simulink model "heli_quanser_base_MC"  (R2025a)
settings: Solver=FixedStepAuto  StartTime=0.0  StopTime=15  FixedStep=0.001  RelTol=1e-3  EnableMultiTasking=on
values from neighbouring files (symbols this model uses):
  theta_0 = -40.5*pi/180    (= -0.706858347058)    [setup_heli_2d_base.m]
  Ts = 0.001    [setup_heli_2d_base.m]
  VMAX_UPM_P = 24    [setup_heli_2d_base.m]
  VMAX_UPM_Y = 15    [setup_heli_2d_base.m]
undefined symbols (not defined in the file or in its folder): B_p, B_y, g, J_eq_p, J_eq_y, K_pp, K_py, K_yp, K_yy, l_cm, m_heli
libraries: simulink x2, simulink_extras x1
settings Model: Creator=Jorge Romero  LastModifiedBy=440G5
settings SolverCC: AlgebraicLoopSolver=TrustRegion
settings DataIOCC: LimitDataPoints=on  SaveFormat=Array  ReturnWorkspaceOutputs=off
settings OptimizationCC: ExpressionDepthLimit=2147483647.0  LifeSpan=inf
settings DebuggingCC: UnderspecifiedInitializationDetection=Classic  MergeDetectMultiDrivingBlocksExec=none  SolverPrmCheckMsg=warning  UnconnectedInputMsg=warning  UnconnectedOutputMsg=warning  UnconnectedLineMsg=warning  StateNameClashWarn=warning  SFUnexpectedBacktrackingDiag=warning  SFNoUnconditionalDefaultTransitionDiag=warning  SFExecutionAtInitializationDiag=none  ArithmeticOperatorsInVariantConditions=warning
settings HardwareCC: ProdBitPerPointer=32.0  ProdBitPerSizeT=32.0  ProdBitPerPtrDiffT=32.0  ProdLargestAtomicFloat=None  ProdIntDivRoundTo=Undefined  ProdEndianess=Unspecified  ProdWordSize=32.0  ProdHWDeviceType=32-bit Generic
settings ModelReferenceCC: EnableRefExpFcnMdlSchedulingChecks=on  PropagateSignalLabelsOutOfModel=off
settings SFSimCC: SimUseLocalCustomCode=off  CustomCodeUndefinedFunction=UseInterfaceOnly
settings RTWCC: RTWUseLocalCustomCode=off  GPUComputeCapability=3.5  DLArmComputeVersion=19.05
settings CodeAppCC: StateflowObjectComments=on
settings GRTTargetCC: TargetLangStandard=C89/C90 (ANSI)
settings ConfigComp: CovMetricSettings=dw  CovSaveCumulativeToWorkspaceVar=on  CovSaveSingleToWorkspaceVar=on  CovExternalEMLEnable=off

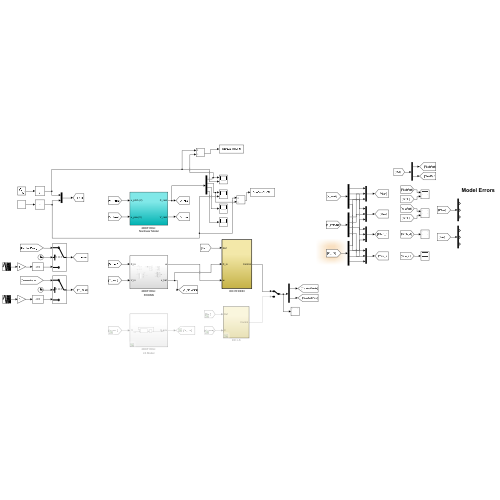
[thumbnail: Simulink's stored preview of the top-level diagram]
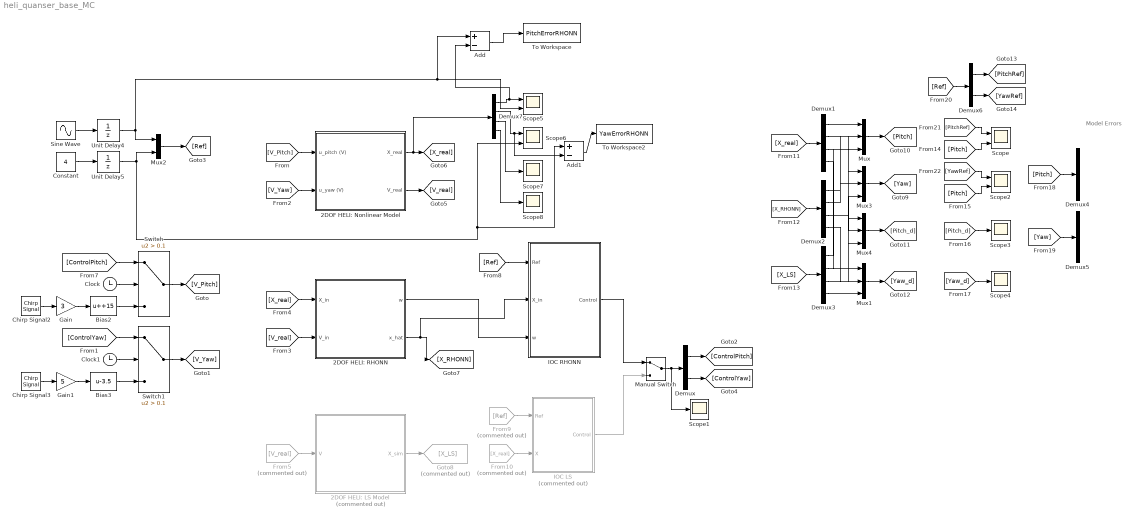
== system heli_quanser_base_MC ==
  note: Model Errors
  2DOF HELI: LS Model : Subsystem  Commented=on
  2DOF HELI: Nonlinear Model : Subsystem
  2DOF HELI: RHONN : Subsystem
  Add : Sum  Inputs=+-
  Add1 : Sum  Inputs=+-
  Bias2 : Bias  Bias=+15  SaturateOnIntegerOverflow=off
  Bias3 : Bias  Bias=-3.5  SaturateOnIntegerOverflow=off
  Chirp Signal2 : simulink/Sources/Chirp Signal  f1=0.08  T=10  f2=1
  Chirp Signal3 : simulink/Sources/Chirp Signal  f1=0.05  T=100  f2=1
  Clock : Clock
      settings: Decimation=5
  Clock1 : Clock
      settings: Decimation=5
  Constant : Constant  Value=4
  Demux : Demux  Outputs=2
  Demux{1..3,7} (4 alike) : Demux
  Demux4 : Demux  Outputs=3
  Demux5 : Demux  Outputs=3
  Demux6 : Demux  Outputs=2
  From10 : From  Commented=on  GotoTag=X_real
  From5 : From  Commented=on  GotoTag=V_real
  From9 : From  Commented=on  GotoTag=Ref
  Gain : Gain  Gain=3
  Gain1 : Gain  Gain=5
  Goto8 : Goto  Commented=on  GotoTag=X_LS
  IOC LS : Subsystem  Commented=on  TreatAsAtomicUnit=on
  IOC RHONN : Subsystem  TreatAsAtomicUnit=on
  Manual Switch : ManualSwitch
  Mux{,1,3..4} (4 alike) : Mux  Inputs=3
  Mux2 : Mux  Inputs=2
  Scope{,2,5..6} (4 alike) : Scope  NumInputPorts=2
      Scope settings: ActiveDisplayYMinimum=-2.2045251175704  ActiveDisplayYMaximum=12.772142587556569
      Scope2 settings: ActiveDisplayYMinimum=-2.2045251175704  ActiveDisplayYMaximum=12.772142587556569
      Scope5 settings: ActiveDisplayYMinimum=-1.4995166148869326  ActiveDisplayYMaximum=1.1943818734120628  DataLoggingVariableName=ScopeData4
      Scope6 settings: ActiveDisplayYMinimum=-31.385745513206732  ActiveDisplayYMaximum=23.73492677473369  DataLoggingVariableName=ScopeData5
  Scope{1,3..4,7..8} (5 alike) : Scope
      Scope1 settings: ActiveDisplayYMinimum=-26.503210929485832  ActiveDisplayYMaximum=16.085993128612095  DataLoggingVariableName=ScopeData14
      Scope3 settings: DataLoggingVariableName=ScopeData2
      Scope4 settings: DataLoggingVariableName=ScopeData3
      Scope7 settings: ActiveDisplayYMinimum=-2.2729284352396681  ActiveDisplayYMaximum=0.21801617430591014  DataLoggingVariableName=ScopeData6
      Scope8 settings: ActiveDisplayYMinimum=-1  ActiveDisplayYMaximum=1  DataLoggingVariableName=ScopeData7
  Sine Wave : Sin  Amplitude=0.45  SampleTime=0
  Switch : Switch  Criteria=u2 > Threshold  Threshold=0.1  SaturateOnIntegerOverflow=off  InputSameDT=off
  Switch1 : Switch  Criteria=u2 > Threshold  Threshold=0.1  SaturateOnIntegerOverflow=off  InputSameDT=off
  To Workspace : ToWorkspace  VariableName=PitchErrorRHONN  SaveFormat=Timeseries  SampleTime=-1
  To Workspace2 : ToWorkspace  VariableName=YawErrorRHONN  SaveFormat=Timeseries  SampleTime=-1
  Unit Delay4 : UnitDelay  SampleTime=-1  HasFrameUpgradeWarning=on
  Unit Delay5 : UnitDelay  SampleTime=-1  HasFrameUpgradeWarning=on
  wires:
  Gain/1 -> Bias2/1
  Bias2/1 -> Switch/3
  Chirp Signal2/1 -> Gain/1
  [ControlPitch] -> Switch/1
  Clock/1 -> Switch/2
  Bias3/1 -> Switch1/3
  Gain1/1 -> Bias3/1
  Clock1/1 -> Switch1/2
  Chirp Signal3/1 -> Gain1/1
  [ControlYaw] -> Switch1/1
  Switch/1 -> [V_Pitch]
  Switch1/1 -> [V_Yaw]
  [V_Pitch] -> 2DOF HELI: Nonlinear Model/1(u_pitch (V))
  [V_Yaw] -> 2DOF HELI: Nonlinear Model/2(u_yaw (V))
  From5/1 -> 2DOF HELI: LS Model/1(" V")
  IOC LS/1(Control) -> Manual Switch/2
  From9/1 -> IOC LS/1(Ref)
  Unit Delay4/1 -> Add/1, Scope5/2, Mux2/1
  Mux2/1 -> [Ref]
  Manual Switch/1 -> Scope1/1, Demux/1
  Demux/1 -> [ControlPitch]
  Demux/2 -> [ControlYaw]
  2DOF HELI: Nonlinear Model/2(V_real) -> [V_real]
  2DOF HELI: Nonlinear Model/1(X_real) -> Demux7/1, [X_real]
  From10/1 -> IOC LS/2(X)
  2DOF HELI: LS Model/1(X_sim) -> Goto8/1
  [X_RHONN] -> Demux2/1
  [X_real] -> Demux1/1
  [X_LS] -> Demux3/1
  Demux1/1 -> Mux/1
  Demux2/1 -> Mux/2
  Demux3/1 -> Mux/3
  Demux1/4 -> Mux1/1
  Demux2/4 -> Mux1/2
  Demux3/4 -> Mux1/3
  Demux1/2 -> Mux3/1
  Demux2/2 -> Mux3/2
  Demux3/2 -> Mux3/3
  Demux1/3 -> Mux4/1
  Demux2/3 -> Mux4/2
  Demux3/3 -> Mux4/3
  Mux/1 -> [Pitch]
  Mux3/1 -> [Yaw]
  Mux4/1 -> [Pitch_d]
  Mux1/1 -> [Yaw_d]
  [Pitch] -> Scope/2
  [Pitch_d] -> Scope3/1
  [Yaw_d] -> Scope4/1
  [Pitch] -> Demux4/1
  [Yaw] -> Demux5/1
  [Ref] -> Demux6/1
  [PitchRef] -> Scope/1
  [YawRef] -> Scope2/1
  [Pitch] -> Scope2/2
  Demux6/1 -> [PitchRef]
  Demux6/2 -> [YawRef]
  2DOF HELI: RHONN/2(x_hat) -> IOC RHONN/2(X_in), [X_RHONN]
  [X_real] -> 2DOF HELI: RHONN/1(X_in)
  [V_real] -> 2DOF HELI: RHONN/2(V_in)
  2DOF HELI: RHONN/1(w) -> IOC RHONN/3(w)
  IOC RHONN/1(Control) -> Manual Switch/1
  [Ref] -> IOC RHONN/1(Ref)
  Sine Wave/1 -> Unit Delay4/1
  Constant/1 -> Unit Delay5/1
  Demux7/1 -> Add/2, Scope5/1
  Demux7/2 -> Add1/2, Scope6/1
  Demux7/3 -> Scope7/1
  Demux7/4 -> Scope8/1
  Add/1 -> To Workspace/1
  Unit Delay5/1 -> Mux2/2, Scope6/2, Add1/1
  Add1/1 -> To Workspace2/1

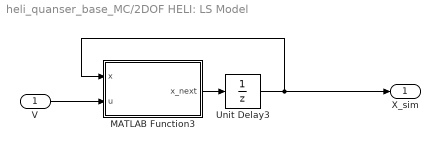
== system heli_quanser_base_MC/2DOF HELI: LS Model ==
  " V" : Inport
  MATLAB Function3 : MATLAB Function  TreatAsAtomicUnit=on
  Unit Delay3 : UnitDelay  InitialCondition=|  SampleTime=-1  HasFrameUpgradeWarning=on
      | [ -40.5*pi/180;
      |         0 ;
      |         0 ;
      |         0 ];
  X_sim : Outport
  wires:
  Unit Delay3/1 -> X_sim/1, MATLAB Function3/1(x)
  MATLAB Function3/1(x_next) -> Unit Delay3/1
  " V"/1 -> MATLAB Function3/2(u)

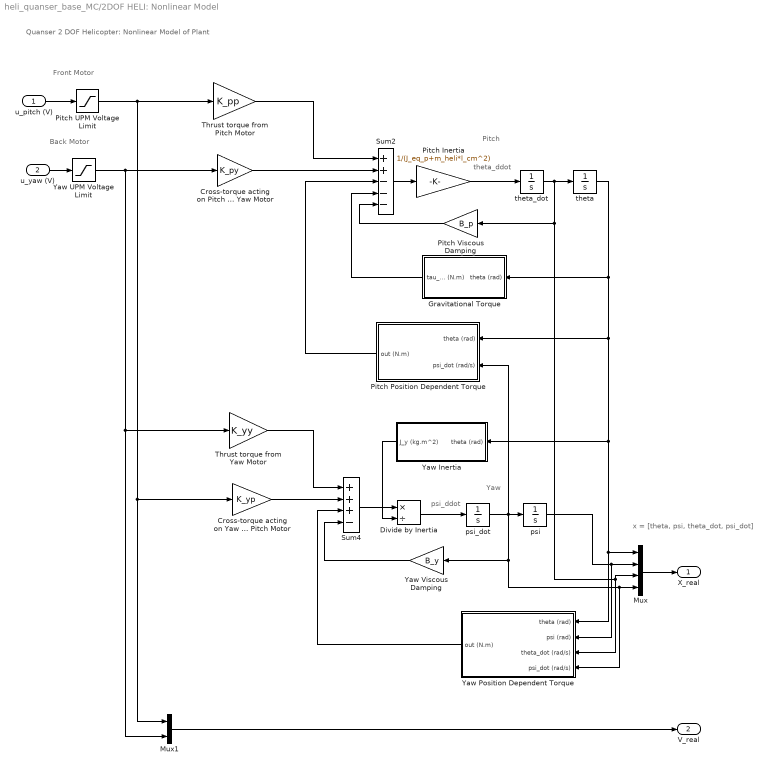
== system heli_quanser_base_MC/2DOF HELI: Nonlinear Model ==
  note: Back Motor
  note: Front Motor
  note: x = [theta, psi, theta_dot, psi_dot]
  note: Quanser 2 DOF Helicopter: Nonlinear Model of Plant
  note: theta_ddot
  note: psi_ddot
  note: Pitch
  note: Yaw
  u_pitch (V) : Inport
  u_yaw (V) : Inport  Port=2
  Cross-torque acting on Pitch from Yaw Motor : Gain  Gain=K_py
  Cross-torque acting on Yaw from Pitch Motor : Gain  Gain=K_yp
  Divide by Inertia : Product  Inputs=*/
  Gravitational Torque : Subsystem
  Mux : Mux
  Mux1 : Mux  Inputs=2
  Pitch Inertia : Gain  Gain=1/(J_eq_p+m_heli*l_cm^2)
  Pitch Position Dependent Torque : Subsystem  AncestorBlock=heli_2d_lib/2DOF Helicopter: Nonlinear Model/Yaw Nonlinear Element
  Pitch UPM Voltage Limit : Saturate  UpperLimit=VMAX_UPM_P  LowerLimit=- VMAX_UPM_P
  Pitch Viscous Damping : Gain  Gain=B_p
  Sum2 : Sum  Inputs=++---
  Sum4 : Sum  Inputs=+++-
  Thrust torque from Pitch Motor : Gain  Gain=K_pp
  Thrust torque from Yaw Motor : Gain  Gain=K_yy
  Yaw Inertia : Subsystem
  Yaw Position Dependent Torque : Subsystem
  Yaw UPM Voltage Limit : Saturate  UpperLimit=VMAX_UPM_Y  LowerLimit=- VMAX_UPM_Y
  Yaw Viscous Damping : Gain  Gain=B_y
  psi : Integrator
  psi_dot : Integrator
  theta : Integrator  InitialCondition=theta_0  LimitOutput=on  UpperSaturationLimit=40.5*pi/180  LowerSaturationLimit=-40.5*pi/180
  theta_dot : Integrator
  X_real : Outport
  V_real : Outport  Port=2
  wires:
  Pitch Position Dependent Torque/1(out (N.m)) -> Sum2/3
  Gravitational Torque/1(tau_g (N.m)) -> Sum2/4
  Pitch Viscous Damping/1 -> Sum2/5
  Cross-torque acting on Pitch from Yaw Motor/1 -> Sum2/2
  Thrust torque from Pitch Motor/1 -> Sum2/1
  Yaw Inertia/1(J_y (kg.m^2)) -> Divide by Inertia/2
  Divide by Inertia/1 -> psi_dot/1
  Sum4/1 -> Divide by Inertia/1
  Yaw Position Dependent Torque/1(out (N.m)) -> Sum4/3
  Yaw Viscous Damping/1 -> Sum4/4
  psi/1 -> Yaw Position Dependent Torque/2(psi (rad)), Mux/2
  Mux1/1 -> V_real/1
  Yaw UPM Voltage Limit/1 -> Thrust torque from Yaw Motor/1, Mux1/2, Cross-torque acting on Pitch from Yaw Motor/1
  Pitch UPM Voltage Limit/1 -> Mux1/1, Cross-torque acting on Yaw from Pitch Motor/1, Thrust torque from Pitch Motor/1
  Mux/1 -> X_real/1
  theta/1 -> Gravitational Torque/1(theta (rad)), Pitch Position Dependent Torque/1(theta (rad)), Yaw Position Dependent Torque/1(theta (rad)), Mux/1, Yaw Inertia/1(theta (rad))
  Sum2/1 -> Pitch Inertia/1
  Pitch Inertia/1 -> theta_dot/1
  theta_dot/1 -> Pitch Viscous Damping/1, Yaw Position Dependent Torque/3(theta_dot (rad/s)), Mux/3, theta/1
  Thrust torque from Yaw Motor/1 -> Sum4/1
  Cross-torque acting on Yaw from Pitch Motor/1 -> Sum4/2
  psi_dot/1 -> Yaw Viscous Damping/1, Yaw Position Dependent Torque/4(psi_dot (rad/s)), Mux/4, Pitch Position Dependent Torque/2(psi_dot (rad/s)), psi/1
  u_pitch (V)/1 -> Pitch UPM Voltage Limit/1
  u_yaw (V)/1 -> Yaw UPM Voltage Limit/1

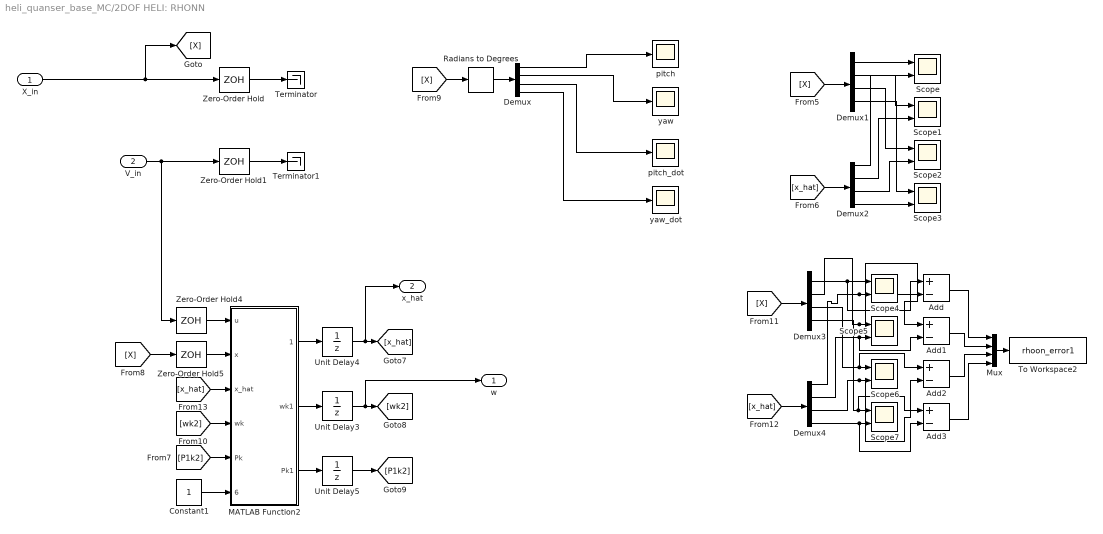
== system heli_quanser_base_MC/2DOF HELI: RHONN ==
  X_in : Inport
  V_in : Inport  Port=2
  Add{,1..3} (4 alike) : Sum  Inputs=+-
  Constant1 : Constant
  Demux{,1..4} (5 alike) : Demux
      Demux settings: DisplayOption=none
  MATLAB Function2 : MATLAB Function  TreatAsAtomicUnit=on
  Mux : Mux
  Radians to Degrees : simulink_extras/Transformations/Radians to Degrees
  Scope{,1..7} (8 alike) : Scope  NumInputPorts=2
      Scope settings: ActiveDisplayYMinimum=-0.76823581059186186  ActiveDisplayYMaximum=-0.420304444530908  DataLoggingVariableName=ScopeData25
      Scope1 settings: ActiveDisplayYMinimum=-4.0467602217743632  ActiveDisplayYMaximum=10.170477768659628  DataLoggingVariableName=ScopeData26
      Scope2 settings: ActiveDisplayYMinimum=-2.8805560704362327  ActiveDisplayYMaximum=0.42254717438739869  DataLoggingVariableName=ScopeData15
      Scope3 settings: ActiveDisplayYMinimum=-0.60551922567826943  ActiveDisplayYMaximum=1.2844796238730485  DataLoggingVariableName=ScopeData27
      Scope4 settings: ActiveDisplayYMinimum=-1.1415026108241673  ActiveDisplayYMaximum=0.12683362342490745  DataLoggingVariableName=ScopeData21
      Scope5 settings: ActiveDisplayYMinimum=0.00065987107501674913  ActiveDisplayYMaximum=4.6512841717291593  DataLoggingVariableName=ScopeData22
      Scope6 settings: ActiveDisplayYMinimum=-136.21614176214669  ActiveDisplayYMaximum=1171.9792706431781  DataLoggingVariableName=ScopeData23
      Scope7 settings: ActiveDisplayYMinimum=-1.1741616508954156  ActiveDisplayYMaximum=1.4302738530662835  DataLoggingVariableName=ScopeData24
  Terminator : Terminator
  Terminator1 : Terminator
  To Workspace2 : ToWorkspace  VariableName=rhoon_error1  SaveFormat=Timeseries  SampleTime=-1
  Unit Delay3 : UnitDelay  InitialCondition=zeros(16,1)  SampleTime=-1  HasFrameUpgradeWarning=on
  Unit Delay4 : UnitDelay  InitialCondition=[0;0;0;0]  SampleTime=-1  HasFrameUpgradeWarning=on
  Unit Delay5 : UnitDelay  InitialCondition=zeros(4,4,4)  SampleTime=-1  HasFrameUpgradeWarning=on
  Zero-Order Hold4 : ZeroOrderHold  SampleTime=-1
  Zero-Order Hold5 : ZeroOrderHold  SampleTime=-1
  Zero-Order Hold : ZeroOrderHold  SampleTime=Ts
  Zero-Order Hold1 : ZeroOrderHold  SampleTime=Ts
  pitch : Scope
      settings: TimeSpan=30  ActiveDisplayYMinimum=-81.99762  ActiveDisplayYMaximum=9.11085  DataLoggingVariableName=ScopeData28
  pitch_dot : Scope
      settings: TimeSpan=30  ActiveDisplayYMinimum=-48.65452  ActiveDisplayYMaximum=62.46494  DataLoggingVariableName=ScopeData18
  yaw : Scope
      settings: TimeSpan=30  ActiveDisplayYMinimum=-31.83031  ActiveDisplayYMaximum=286.47281  DataLoggingVariableName=ScopeData19
  yaw_dot : Scope
      settings: TimeSpan=30  ActiveDisplayYMinimum=-83.27416  ActiveDisplayYMaximum=83.72639  DataLoggingVariableName=ScopeData20
  w : Outport
  x_hat : Outport  Port=2
  wires:
  Demux1/2 -> Scope1/1
  Add2/1 -> Mux/3
  [x_hat] -> Demux2/1
  [P1k2] -> MATLAB Function2/5(Pk)
  Demux3/3 -> Add2/1, Scope6/1
  Demux/3 -> pitch_dot/1
  Demux2/3 -> Scope2/2
  MATLAB Function2/1(x_hat_k1) -> Unit Delay4/1
  [X] -> Radians to Degrees/1
  [wk2] -> MATLAB Function2/4(wk)
  [X] -> Demux1/1
  Demux2/4 -> Scope3/2
  Radians to Degrees/1 -> Demux/1
  Demux2/1 -> Scope/2
  Demux2/2 -> Scope1/2
  Zero-Order Hold5/1 -> MATLAB Function2/2(x)
  [x_hat] -> MATLAB Function2/3(x_hat)
  Demux4/1 -> Add/2, Scope4/2
  [x_hat] -> Demux4/1
  Demux3/2 -> Add1/1, Scope5/1
  Unit Delay3/1 -> w/1, [wk2]
  MATLAB Function2/3(Pk1) -> Unit Delay5/1
  Mux/1 -> To Workspace2/1
  Demux/2 -> yaw/1
  [X] -> Zero-Order Hold5/1
  Demux1/3 -> Scope2/1
  Demux4/3 -> Add2/2, Scope6/2
  Demux3/1 -> Add/1, Scope4/1
  Zero-Order Hold1/1 -> Terminator1/1
  Demux1/4 -> Scope3/1
  Add1/1 -> Mux/2
  Demux/1 -> pitch/1
  MATLAB Function2/2(wk1) -> Unit Delay3/1
  X_in/1 -> [X], Zero-Order Hold/1
  Demux4/2 -> Scope5/2, Add1/2
  Unit Delay5/1 -> [P1k2]
  Unit Delay4/1 -> x_hat/1, [x_hat]
  Constant1/1 -> MATLAB Function2/6(basis_id)
  Zero-Order Hold/1 -> Terminator/1
  Demux3/4 -> Add3/1, Scope7/1
  Demux1/1 -> Scope/1
  Zero-Order Hold4/1 -> MATLAB Function2/1(u)
  [X] -> Demux3/1
  V_in/1 -> Zero-Order Hold1/1, Zero-Order Hold4/1
  Add/1 -> Mux/1
  Demux4/4 -> Add3/2, Scope7/2
  Add3/1 -> Mux/4
  Demux/4 -> yaw_dot/1

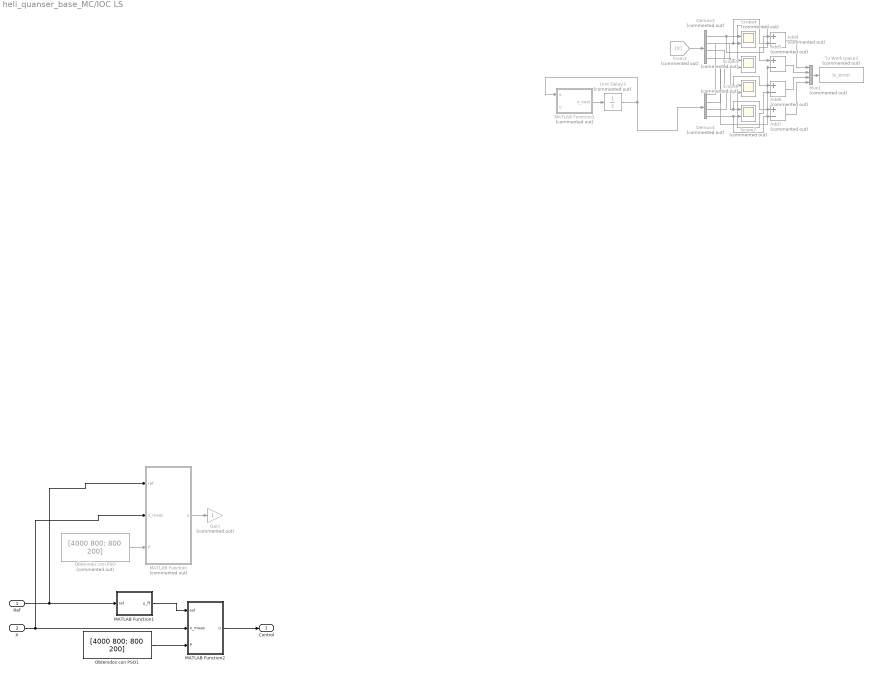
== system heli_quanser_base_MC/IOC LS ==
  Ref : Inport
  X : Inport  Port=2
  Add{4..7} (4 alike) : Sum  Commented=on  Inputs=+-
  Demux3 : Demux  Commented=on
  Demux4 : Demux  Commented=on
  From3 : From  Commented=on  GotoTag=X
  Gain : Gain  Commented=on
  MATLAB Function : MATLAB Function  Commented=on  TreatAsAtomicUnit=on
  MATLAB Function1 : MATLAB Function  TreatAsAtomicUnit=on
  MATLAB Function2 : MATLAB Function  TreatAsAtomicUnit=on
  MATLAB Function3 : MATLAB Function  Commented=on  TreatAsAtomicUnit=on
  Mux1 : Mux  Commented=on
  Obtenidos con PSO : Constant  Commented=on  Value=[4000 800; 800 200]
  Obtenidos con PSO1 : Constant  Value=[4000 800; 800 200]
  Scope{4..7} (4 alike) : Scope  Commented=on  NumInputPorts=2
      Scope4 settings: ActiveDisplayYMinimum=-0.78569456230161683  ActiveDisplayYMaximum=0.0026675901375168704  DataLoggingVariableName=ScopeData8
      Scope5 settings: ActiveDisplayYMinimum=-0.45463938909370377  ActiveDisplayYMaximum=4.0917545018433348  DataLoggingVariableName=ScopeData9
      Scope6 settings: ActiveDisplayYMinimum=-0.49237684754972044  ActiveDisplayYMaximum=0.55901528153260716  DataLoggingVariableName=ScopeData10
      Scope7 settings: ActiveDisplayYMinimum=-0.14622878783376417  ActiveDisplayYMaximum=1.3160590905038778  DataLoggingVariableName=ScopeData11
  To Workspace3 : ToWorkspace  Commented=on  VariableName=ls_error  SaveFormat=Timeseries  SampleTime=-1
  Unit Delay3 : UnitDelay  Commented=on  InitialCondition=|  SampleTime=-1  HasFrameUpgradeWarning=on
      | [ -40.5*pi/180 ;
      |         0 ;
      |         0 ;
      |         0 ];
  Control : Outport
  wires:
  MATLAB Function3/1(x_next) -> Unit Delay3/1
  Add6/1 -> Mux1/3
  Add4/1 -> Mux1/1
  Demux4/4 -> Add7/2, Scope7/2
  From3/1 -> Demux3/1
  Demux3/1 -> Add4/1, Scope4/1
  Demux3/4 -> Add7/1, Scope7/1
  Demux3/2 -> Add5/1, Scope5/1
  Mux1/1 -> To Workspace3/1
  Add7/1 -> Mux1/4
  Demux3/3 -> Add6/1, Scope6/1
  Add5/1 -> Mux1/2
  Demux4/3 -> Add6/2, Scope6/2
  Demux4/2 -> Scope5/2, Add5/2
  Unit Delay3/1 -> Demux4/1, MATLAB Function3/1(x)
  Demux4/1 -> Add4/2, Scope4/2
  MATLAB Function/1(u) -> Gain/1
  X/1 -> MATLAB Function/2(x_meas), MATLAB Function2/2(x_meas)
  Obtenidos con PSO/1 -> MATLAB Function/3(P)
  Ref/1 -> MATLAB Function/1(ref), MATLAB Function1/1(ref)
  MATLAB Function1/1(u_ff) -> MATLAB Function2/1(ref)
  Obtenidos con PSO1/1 -> MATLAB Function2/3(P)
  MATLAB Function2/1(u) -> Control/1

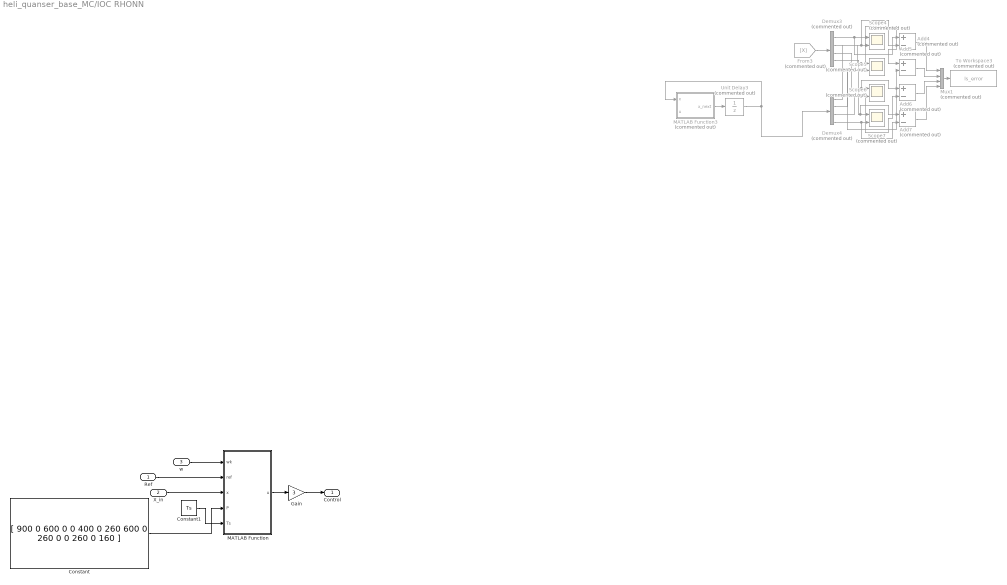
== system heli_quanser_base_MC/IOC RHONN ==
  Ref : Inport
  X_in : Inport  Port=2
  w : Inport  Port=3
  Add{4..7} (4 alike) : Sum  Commented=on  Inputs=+-
  Constant : Constant  Value=|  VectorParams1D=off
      | [ 900   0  600   0
      |     0 400    0 260
      |   600   0  260   0
      |     0 260    0 160 ]
  Constant1 : Constant  Value=Ts
  Demux3 : Demux  Commented=on
  Demux4 : Demux  Commented=on
  From3 : From  Commented=on  GotoTag=X
  Gain : Gain  Gain=3
  MATLAB Function : MATLAB Function  TreatAsAtomicUnit=on  SystemSampleTime=0.001
  MATLAB Function3 : MATLAB Function  Commented=on  TreatAsAtomicUnit=on
  Mux1 : Mux  Commented=on
  Scope{4..7} (4 alike) : Scope  Commented=on  NumInputPorts=2
      Scope4 settings: ActiveDisplayYMinimum=-0.78569456230161683  ActiveDisplayYMaximum=0.0026675901375168704  DataLoggingVariableName=ScopeData8
      Scope5 settings: ActiveDisplayYMinimum=-0.45463938909370377  ActiveDisplayYMaximum=4.0917545018433348  DataLoggingVariableName=ScopeData9
      Scope6 settings: ActiveDisplayYMinimum=-0.49237684754972044  ActiveDisplayYMaximum=0.55901528153260716  DataLoggingVariableName=ScopeData10
      Scope7 settings: ActiveDisplayYMinimum=-0.14622878783376417  ActiveDisplayYMaximum=1.3160590905038778  DataLoggingVariableName=ScopeData11
  To Workspace3 : ToWorkspace  Commented=on  VariableName=ls_error  SaveFormat=Timeseries  SampleTime=-1
  Unit Delay3 : UnitDelay  Commented=on  InitialCondition=|  SampleTime=-1  HasFrameUpgradeWarning=on
      | [ -40.5*pi/180 ;
      |         0 ;
      |         0 ;
      |         0 ];
  Control : Outport
  wires:
  MATLAB Function3/1(x_next) -> Unit Delay3/1
  Add6/1 -> Mux1/3
  Add4/1 -> Mux1/1
  Demux4/4 -> Add7/2, Scope7/2
  From3/1 -> Demux3/1
  Demux3/1 -> Add4/1, Scope4/1
  Demux3/4 -> Add7/1, Scope7/1
  Demux3/2 -> Add5/1, Scope5/1
  Mux1/1 -> To Workspace3/1
  Add7/1 -> Mux1/4
  Demux3/3 -> Add6/1, Scope6/1
  Add5/1 -> Mux1/2
  Demux4/3 -> Add6/2, Scope6/2
  Demux4/2 -> Scope5/2, Add5/2
  Unit Delay3/1 -> Demux4/1, MATLAB Function3/1(x)
  Demux4/1 -> Add4/2, Scope4/2
  w/1 -> MATLAB Function/1(wk)
  Ref/1 -> MATLAB Function/2(ref)
  X_in/1 -> MATLAB Function/3(x)
  Constant/1 -> MATLAB Function/4(P)
  Constant1/1 -> MATLAB Function/5(Ts)
  MATLAB Function/1(u) -> Gain/1
  Gain/1 -> Control/1

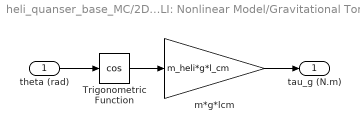
== system heli_quanser_base_MC/2DOF HELI: Nonlinear Model/Gravitational Torque ==
  theta (rad) : Inport
  Trigonometric Function : Trigonometry  Operator=cos  OutputSignalType=real
  m*g*lcm : Gain  Gain=m_heli*g*l_cm
  tau_g (N.m) : Outport
  wires:
  m*g*lcm/1 -> tau_g (N.m)/1
  theta (rad)/1 -> Trigonometric Function/1
  Trigonometric Function/1 -> m*g*lcm/1

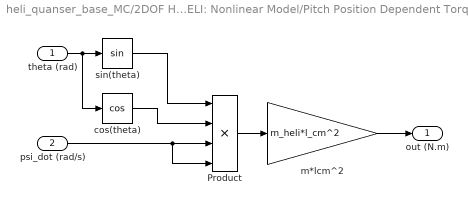
== system heli_quanser_base_MC/2DOF HELI: Nonlinear Model/Pitch Position Dependent Torque ==
  theta (rad) : Inport
  psi_dot (rad/s) : Inport  Port=2
  Product : Product  Inputs=4  RndMeth=Zero
  cos(theta) : Trigonometry  Operator=cos  OutputSignalType=real
  m*lcm^2 : Gain  Gain=m_heli*l_cm^2
  sin(theta) : Trigonometry  OutputSignalType=real
  out (N.m) : Outport
  wires:
  psi_dot (rad/s)/1 -> Product/4, Product/3
  theta (rad)/1 -> cos(theta)/1, sin(theta)/1
  Product/1 -> m*lcm^2/1
  sin(theta)/1 -> Product/1
  cos(theta)/1 -> Product/2
  m*lcm^2/1 -> out (N.m)/1

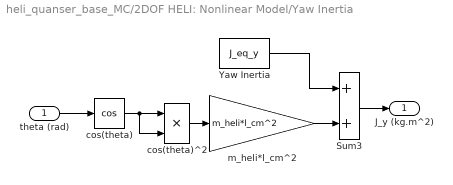
== system heli_quanser_base_MC/2DOF HELI: Nonlinear Model/Yaw Inertia ==
  theta (rad) : Inport
  Sum3 : Sum
  Yaw Inertia : Constant  Value=J_eq_y
  cos(theta) : Trigonometry  Operator=cos  OutputSignalType=real
  cos(theta)^2 : Product  RndMeth=Zero
  m_heli*l_cm^2 : Gain  Gain=m_heli*l_cm^2
  J_y (kg.m^2) : Outport
  wires:
  cos(theta)/1 -> cos(theta)^2/2, cos(theta)^2/1
  Sum3/1 -> J_y (kg.m^2)/1
  theta (rad)/1 -> cos(theta)/1
  m_heli*l_cm^2/1 -> Sum3/2
  Yaw Inertia/1 -> Sum3/1
  cos(theta)^2/1 -> m_heli*l_cm^2/1

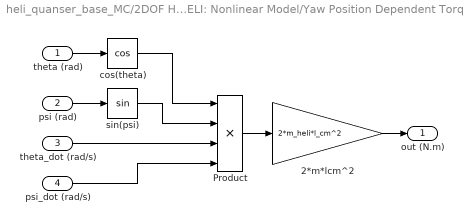
== system heli_quanser_base_MC/2DOF HELI: Nonlinear Model/Yaw Position Dependent Torque ==
  theta (rad) : Inport
  psi (rad) : Inport  Port=2
  theta_dot (rad/s) : Inport  Port=3
  psi_dot (rad/s) : Inport  Port=4
  2*m*lcm^2 : Gain  Gain=2*m_heli*l_cm^2
  Product : Product  Inputs=4  RndMeth=Zero
  cos(theta) : Trigonometry  Operator=cos  OutputSignalType=real
  sin(psi) : Trigonometry  OutputSignalType=real
  out (N.m) : Outport
  wires:
  2*m*lcm^2/1 -> out (N.m)/1
  psi_dot (rad/s)/1 -> Product/4
  theta_dot (rad/s)/1 -> Product/3
  sin(psi)/1 -> Product/2
  cos(theta)/1 -> Product/1
  Product/1 -> 2*m*lcm^2/1
  theta (rad)/1 -> cos(theta)/1
  psi (rad)/1 -> sin(psi)/1

== matlab function heli_quanser_base_MC/2DOF HELI: RHONN/MATLAB Function2 ==
  data: u input; x input; x_hat input; wk input; Pk input; x_hat_k1 output; wk1 output; Pk1 output; basis_id input
function [x_hat_k1, wk1, Pk1] = rhonn_rotary(u, x, x_hat, wk, Pk, basis_id)
% RHONN para heli 2DOF
% Orden de estados que estás usando:
%   x = [pitch; yaw; pitch_dot; yaw_dot]
%
% Entradas:
%   u    : [2x1] (pero aceptamos 1x1 y lo completamos)
%   x    : [4x1]
%   x_hat: [4x1] (no lo usamos mucho aquí, pero lo dejas igual)
%   wk   : [16x1]
%   Pk   : [4x4x4]
%   basis_id: selector de base
%
% Salidas:
%   x_hat_k1 : [4x1]
%   wk1      : [16x1]
%   Pk1      : [4x4x4]

    %% -------- defaults --------
    if nargin < 7
        basis_id = 1;
    end

    % fijar u a 2x1 SIN crecer arrays
    u_fix = zeros(2,1);
    nu = min(2, numel(u));
    u_fix(1:nu) = u(1:nu);

    % fijar x a 4x1
    x_fix = zeros(4,1);
    nx = min(4, numel(x));
    x_fix(1:nx) = x(1:nx);

    % fijar wk
    wk_fix = zeros(16,1);
    nw = min(16, numel(wk));
    wk_fix(1:nw) = wk(1:nw);

    % fijar Pk
    Pk1 = Pk;

    %% ganancias de entrada (mismas que traías)
    w_u2 = [0.15; 0.00];   % para u1 → pitch_dot
    w_u4 = [0.00; 0.15];   % para u2 → yaw_dot

    Q = eye(4)*5e3;
    Rm = 6e3;   % (este R es de medición, no el del control)

    %% -------- base no lineal --------
    a = 0.01;
    switch basis_id
        case 1
            H = tanh(x_fix);
        case 2
            H = 1./(1+exp(-x_fix));
        otherwise
            H = tanh(x_fix);
    end

    %% -------- extraer pesos --------
    w1 = wk_fix( 1: 4);
    w2 = wk_fix( 5: 8);
    w3 = wk_fix( 9:12);
    w4 = wk_fix(13:16);

    %% -------- modelo neuronal (AQUÍ VA TU CAMBIO) --------
    % x1 = pitch
    x1_hat = w1.'*H;
    % x2 = yaw     (ya no recibe u directa)
    x2_hat = w2.'*H;
    % x3 = pitch_dot  (AQUÍ sí recibe u1)
    x3_hat = w3.'*H + w_u2.' * u_fix;
    % x4 = yaw_dot     (AQUÍ sí recibe u2)
    x4_hat = w4.'*H + w_u4.' * u_fix;

    x_hat_k1 = [x1_hat; x2_hat; x3_hat; x4_hat];

    %% -------- EKF por estado (igual que lo tenías) --------
    wk1 = wk_fix;

    e = x_fix - x_hat_k1;   % error por estado

    for i = 1:4
        Pi = Pk(:,:,i);
        Ki = (Pi*H) / (Rm + H.'*Pi*H);

        wi = wk_fix((i-1)*4+1 : i*4);
        wi_new = wi + Ki * e(i);

        Pi_new = Pi - Ki*(H.')*Pi + Q;

        wk1((i-1)*4+1 : i*4) = wi_new;
        Pk1(:,:,i) = Pi_new;
    end
end

== matlab function heli_quanser_base_MC/IOC LS/MATLAB Function1 ==
  data: ref input; u_ff output
function u_ff = trim_from_ls(ref)
    % ref = [pitch; yaw]

    % --- tu modelo ---
    A = [ 1.0000   -0.0000    0.0010    0.0000;
         -0.0000    1.0000    0.0000    0.0010;
         -0.0134   -0.0014    0.9912    0.0148;
         -0.0004   -0.0001    0.0002    0.9973 ];

    B = [ 0.0000   -0.0000;
          0.0000    0.0000;
          0.0013   -0.0025;
          0.0003    0.0007 ];

    c = [ -0.0000;
          -0.0000;
          -0.0281;
          -0.0012 ];

    xref = [ref(1); ref(2); 0; 0];
    rhs  = (eye(4) - A) * xref - c;   % lo que falta para equilibrar

    % B es 4x2, no es cuadrada -> usa pinv
    u_ff = pinv(B) * rhs;             % [up; uy], en VOLTS
end

== matlab function heli_quanser_base_MC/IOC RHONN/MATLAB Function ==
  data: wk input; u output; ref input; x input; P input; Ts input
function u = heli_opt_control(wk, ref, x, P, Ts)
% x   = [theta; psi; dtheta; dpsi]
% ref = [theta_ref; psi_ref]
% P   = 4x4 SPD
% Ts  = sample time [s]

    %#codegen
    assert(isequal(size(wk),[16,1]));
    assert(isequal(size(ref),[2,1]));
    assert(isequal(size(x),[4,1]));
    assert(isequal(size(P),[4,4]));
    assert(isscalar(Ts) && Ts>0);

    % ---- persistentes para integral y derivada discreta de la referencia
    persistent xI ref_prev
    if isempty(xI),      xI = 0;           end        % integral de e_theta
    if isempty(ref_prev),ref_prev = ref;    end

    % ---- parámetros (ajústalos si hace falta)
    Wu   = [0.22 0.50;    % theta_ddot <- [u_p, u_y]
            0.05 0.16];   % psi_ddot   <- [u_p, u_y]
    R    = eye(2);
    u_sat = [24; 15];       % [u_p; u_y] límites
    kI_p  = 0.6;            % GANANCIA INTEGRAL para pitch (empieza en 0.4–0.8)

    % ---- matriz G (u en filas 3 y 4)
    G = [0 0;
         0 0;
         Wu(1,1) Wu(1,2);
         Wu(2,1) Wu(2,2)];

    % ---- referencia + derivada discreta para dtheta_ref
    theta_ref  = ref(1);
    psi_ref    = ref(2);
    dtheta_ref = (ref(1) - ref_prev(1)) / Ts;   % mejor que 0 para seguir seno
    ref_prev   = ref;

    x_des = [theta_ref; psi_ref; dtheta_ref; 0];

    % ---- ley óptima sobre el error de estado
    phi = x - x_des;
    M = (R + 0.5*(G.'*P*G));
    b = (G.'*P*phi);
    u_opt = -0.5 * (M \ b);          % salida “óptima” sin integral

    % ---- integral en pitch (internal-model para eliminar DC)
    e_theta = x(1) - theta_ref;
    xI_new  = xI + Ts * e_theta;
    u_int   = [-kI_p * xI;   0];      % solo en canal de pitch

    u_raw = u_opt + u_int;

    % ---- saturación + anti-windup simple (clamp del integrador)
    u = u_raw;
    if u(1) >  u_sat(1), u(1) =  u_sat(1); end
    if u(1) < -u_sat(1), u(1) = -u_sat(1); end
    if u(2) >  u_sat(2), u(2) =  u_sat(2); end
    if u(2) < -u_sat(2), u(2) = -u_sat(2); end

    % si el canal de pitch está saturado y la integral empuja más a la saturación, congela
    pushing_up   = (u_raw(1) >  u_sat(1)) && (sign(u_int(1)) > 0);
    pushing_down = (u_raw(1) < -u_sat(1)) && (sign(u_int(1)) < 0);
    if ~(pushing_up || pushing_down)
        xI = xI_new;  % actualizar solo si no “empeora” la saturación
    end
end

== matlab function heli_quanser_base_MC/IOC RHONN/MATLAB Function3 ==
  data: x input; u input; x_next output
function x_next = ss_disc_bias(x, u)
%#codegen
% Discrete state-space with bias:
%   x(k+1) = A*x(k) + B*u(k) + c
% Inputs:
%   x : [4x1] current state
%   u : [2x1] input
% Output:
%   x_next : [4x1] next state

% ----- matrices identificadas -----
A = [ 1.0000   -0.0000    0.0010    0.0000;
     -0.0000    1.0000    0.0000    0.0010;
     -0.0134   -0.0014    0.9912    0.0148;
     -0.0004   -0.0001    0.0002    0.9973 ];

B = [ 0.0000   -0.0000;
      0.0000    0.0000;
      0.0013   -0.0025;
      0.0003    0.0007 ];

c = [ -0.0000;
      -0.0000;
      -0.0281;
      -0.0012 ];

% ----- dinámica discreta -----
x_next = A * x + B * u + c;
end

== matlab function heli_quanser_base_MC/2DOF HELI: LS Model/MATLAB Function3 ==
  data: x input; u input; x_next output
function x_next = ss_disc_bias(x, u)
%#codegen
% Discrete state-space with bias:
%   x(k+1) = A*x(k) + B*u(k) + c
% Inputs:
%   x : [4x1] current state
%   u : [2x1] input
% Output:
%   x_next : [4x1] next state

% ----- matrices identificadas -----
A = [ 1.0000   -0.0000    0.0010    0.0000;
     -0.0000    1.0000    0.0000    0.0010;
     -0.0134   -0.0014    0.9912    0.0148;
     -0.0004   -0.0001    0.0002    0.9973 ];

B = [ 0.0000   -0.0000;
      0.0000    0.0000;
      0.0013   -0.0025;
      0.0003    0.0007 ];

c = [ -0.0000;
      -0.0000;
      -0.0281;
      -0.0012 ];

% ----- dinámica discreta -----
x_next = A * x + B * u + c;
end

== matlab function heli_quanser_base_MC/IOC LS/MATLAB Function ==
  data: ref input; u output; x_meas input; P input
function u = inv_opt_ls_2step(ref, x_meas, P)
% ref    : [2x1]  -> referencia de [pitch; yaw]  [rad]
% x_meas : [4x1]  -> estado MEDIDO
% P      : [2x2]  -> pesos (DEBE ser SPD)
% u      : [2x1]  -> voltajes

    % ----- límites físicos -----
    pitch_upper = 40.5*pi/180;
    pitch_lower = -40.5*pi/180;
    yaw_upper   =  pi;     % opcional
    yaw_lower   = -pi;

    % --- modelo identificado ---
    A = [ 1.0000   -0.0000    0.0010    0.0000;
         -0.0000    1.0000    0.0000    0.0010;
         -0.0134   -0.0014    0.9912    0.0148;
         -0.0004   -0.0001    0.0002    0.9973 ];

    B = [ 0.0000   -0.0000;
          0.0000    0.0000;
          0.0013   -0.0025;
          0.0003    0.0007 ];

    c = [ -0.0000;
          -0.0000;
          -0.0281;
          -0.0012 ];

    C = [1 0 0 0;
         0 1 0 0];

    % -------- 1) predicción a 2 pasos CON bias --------
    A2     = A*A;
    x2_hat = A2 * x_meas + (A + eye(4)) * c;
    y2_hat = C * x2_hat;   % [pitch2; yaw2]

    % ----- aplicar límites al modelo -----
    y2_hat(1) = min(max(y2_hat(1), pitch_lower), pitch_upper);
    y2_hat(2) = min(max(y2_hat(2), yaw_lower),   yaw_upper);

    % ----- también limitar la referencia -----
    ref(1) = min(max(ref(1), pitch_lower), pitch_upper);
    ref(2) = min(max(ref(2), yaw_lower),   yaw_upper);

    % ----- efecto del control en k+2 si u(k)=u(k+1) -----
    B2    = A*B + B;     % 4x2
    B_eff = C * B2;      % 2x2

    % -------- 2) pesos --------
    R = 1e-2 * eye(2);   % un poco más grande

    G = B_eff' * P * B_eff;
    S = R + 0.5*G + 1e-9*eye(2);

    % -------- 3) ley IOC --------
    e2 = (y2_hat - ref);      % error proyectado
    u  = -0.5 * ( S \ ( B_eff' * P * e2 ) );
end

== matlab function heli_quanser_base_MC/IOC LS/MATLAB Function2 ==
  data: ref input; u output; x_meas input; P input
function u = fcn(ref, x_meas, P)
%#codegen
% ref    : [2x1]
% x_meas : [4x1]
% P      : [2x2]
% u      : [2x1]

    % asegurar tamaño de salida
    u = zeros(2,1);

    % ----- 1) feedforward desde el modelo LS -----
    u_ff = trim_from_ls_local(ref);

    % ----- 2) control óptimo inverso (2-step) -----
    u_ioc = inv_opt_ls_2step_local(ref, x_meas, P);

    % ----- 3) suma -----
    u = u_ff + u_ioc;

    % ----- 4) saturaciones -----
    % pitch
    if u(1) > 24
        u(1) = 24;
    elseif u(1) < -24
        u(1) = -24;
    end

    % yaw
    if u(2) > 15
        u(2) = 15;
    elseif u(2) < -15
        u(2) = -15;
    end
end

% =====================================================
function u_ff = trim_from_ls_local(ref)
    % modelo identificado
    A = [ 1.0000   -0.0000    0.0010    0.0000;
         -0.0000    1.0000    0.0000    0.0010;
         -0.0134   -0.0014    0.9912    0.0148;
         -0.0004   -0.0001    0.0002    0.9973 ];

    B = [ 0.0000   -0.0000;
          0.0000    0.0000;
          0.0013   -0.0025;
          0.0003    0.0007 ];

    c = [ -0.0000;
          -0.0000;
          -0.0281;
          -0.0012 ];

    % estado de equilibrio que quieres
    xref = [ref(1); ref(2); 0; 0];

    % rhs = (I - A)xref - c
    rhs = (eye(4) - A) * xref - c;

    % resolver B u = rhs por mínimos cuadrados:
    % mejor que pinv para codegen
    BtB = B.' * B;      % 2x2
    BtR = B.' * rhs;    % 2x1
    u_ff = BtB \ BtR;   % 2x1
end

% =====================================================
function u = inv_opt_ls_2step_local(ref, x_meas, P)

    % límites físicos
    pitch_upper = 40.5*pi/180;
    pitch_lower = -40.5*pi/180;
    yaw_upper   =  pi;
    yaw_lower   = -pi;

    % modelo identificado
    A = [ 1.0000   -0.0000    0.0010    0.0000;
         -0.0000    1.0000    0.0000    0.0010;
         -0.0134   -0.0014    0.9912    0.0148;
         -0.0004   -0.0001    0.0002    0.9973 ];

    B = [ 0.0000   -0.0000;
          0.0000    0.0000;
          0.0013   -0.0025;
          0.0003    0.0007 ];

    c = [ -0.0000;
          -0.0000;
          -0.0281;
          -0.0012 ];

    C = [1 0 0 0;
         0 1 0 0];

    % ---- predicción a 2 pasos con bias ----
    A2     = A * A;
    x2_hat = A2 * x_meas + (A + eye(4)) * c;  % x(k+2)
    y2_hat = C * x2_hat;                      % y(k+2)

    % ---- limitar modelo ----
    y2_hat(1) = min(max(y2_hat(1), pitch_lower), pitch_upper);
    y2_hat(2) = min(max(y2_hat(2), yaw_lower),   yaw_upper);

    % ---- limitar referencia ----
    ref(1) = min(max(ref(1), pitch_lower), pitch_upper);
    ref(2) = min(max(ref(2), yaw_lower),   yaw_upper);

    % ---- efecto del control en k+2 si u(k)=u(k+1) ----
    B2    = A * B + B;    % 4x2
    B_eff = C * B2;       % 2x2

    % ---- pesos ----
    R = 1e-2 * eye(2);

    G = B_eff.' * P * B_eff;
    S = R + 0.5 * G + 1e-9 * eye(2);

    e2 = y2_hat - ref;
    u  = -0.5 * ( S \ ( B_eff.' * P * e2 ) );
end

== matlab function heli_quanser_base_MC/IOC LS/MATLAB Function3 ==
  data: x input; u input; x_next output
function x_next = ss_disc_bias(x, u)
%#codegen
% Discrete state-space with bias:
%   x(k+1) = A*x(k) + B*u(k) + c
% Inputs:
%   x : [4x1] current state
%   u : [2x1] input
% Output:
%   x_next : [4x1] next state

% ----- matrices identificadas -----
A = [ 1.0000   -0.0000    0.0010    0.0000;
     -0.0000    1.0000    0.0000    0.0010;
     -0.0134   -0.0014    0.9912    0.0148;
     -0.0004   -0.0001    0.0002    0.9973 ];

B = [ 0.0000   -0.0000;
      0.0000    0.0000;
      0.0013   -0.0025;
      0.0003    0.0007 ];

c = [ -0.0000;
      -0.0000;
      -0.0281;
      -0.0012 ];

% ----- dinámica discreta -----
x_next = A * x + B * u + c;
end
